simulink model "lab1_"  (R2019b)
settings: Solver=VariableStepAuto  StartTime=0.0  StopTime=10.0  RelTol=1e-3
settings Model: Creator=xianyu  LastModifiedBy=xianyu

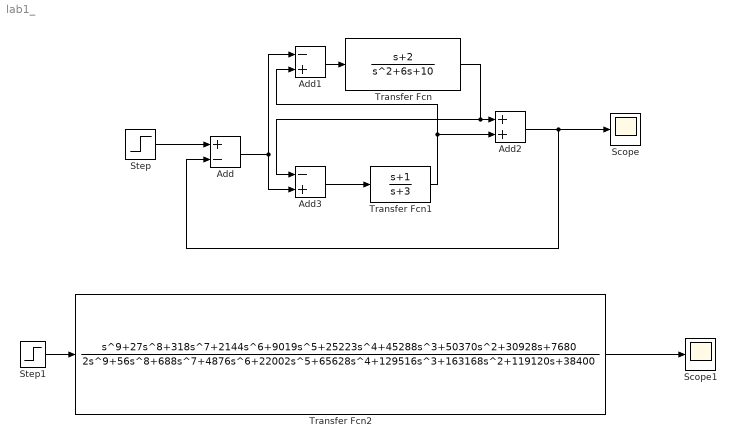
== system lab1_ ==
  Add : Sum  Inputs=+-
  Add1 : Sum  Inputs=-+
  Add2 : Sum
  Add3 : Sum  Inputs=-+
  Scope : Scope
  Scope1 : Scope
  Step : Step  Time=0  SampleTime=0
  Step1 : Step  Time=0  SampleTime=0
  Transfer Fcn : TransferFcn  Numerator=[1 2]  Denominator=[1 6 10]
  Transfer Fcn1 : TransferFcn  Numerator=[1 1]  Denominator=[1 3]
  Transfer Fcn2 : TransferFcn  Numerator=[1 27 318 2144 9019 25223 45288 50370 30928 7680]  Denominator=[2 56 688 4876 22002 65628 129516 163168 119120 38400]
  wires:
  Step/1 -> Add/1
  Add3/1 -> Transfer Fcn1/1
  Add1/1 -> Transfer Fcn/1
  Add2/1 -> Scope/1, Add/2
  Add/1 -> Add1/1, Add3/2
  Transfer Fcn/1 -> Add3/1, Add2/1
  Transfer Fcn1/1 -> Add2/2, Add1/2
  Step1/1 -> Transfer Fcn2/1
  Transfer Fcn2/1 -> Scope1/1
